simulink model "project4"  (R2023b)
settings: Solver=VariableStepAuto  StartTime=0.0  StopTime=10.0  RelTol=1e-3
undefined symbols (not defined in the file or in its folder): Kd, Ki, Kp
settings Model: Creator=mfb36  LastModifiedBy=mfb36

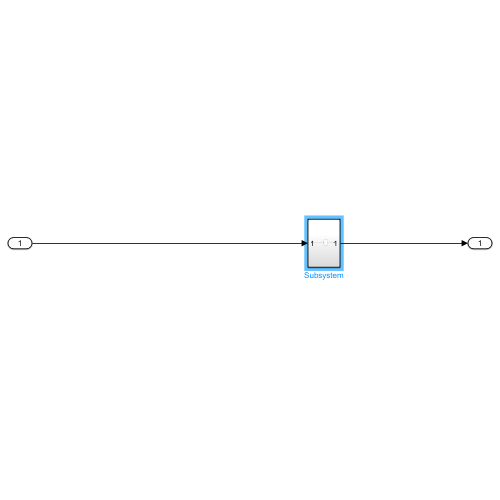
[thumbnail: Simulink's stored preview of the top-level diagram]
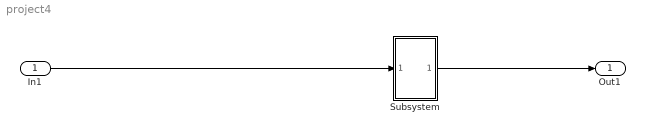
== system project4 ==
  In1 : Inport
  Subsystem : Subsystem
  Out1 : Outport
  wires:
  In1/1 -> Subsystem/1(In1)
  Subsystem/1(Out1) -> Out1/1

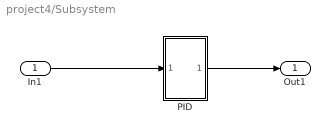
== system project4/Subsystem ==
  In1 : Inport
  PID : Subsystem
  Out1 : Outport
  wires:
  In1/1 -> PID/1(Error)
  PID/1(Control Action) -> Out1/1

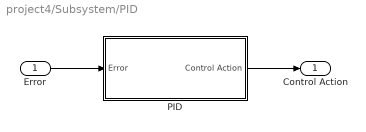
== system project4/Subsystem/PID ==
  Error : Inport
  PID : Subsystem
  Control Action : Outport
  wires:
  Error/1 -> PID/1(Error)
  PID/1(Control Action) -> Control Action/1

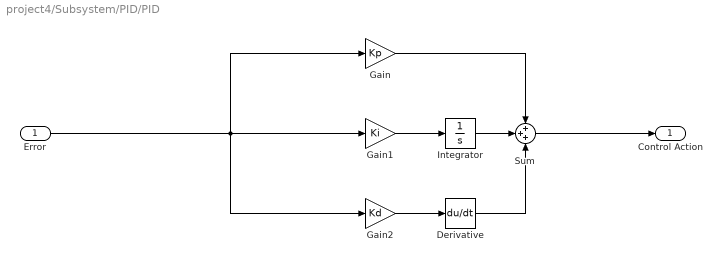
== system project4/Subsystem/PID/PID ==
  Error : Inport
  Derivative : Derivative
  Gain : Gain  Gain=Kp
  Gain1 : Gain  Gain=Ki
  Gain2 : Gain  Gain=Kd
  Integrator : Integrator
  Sum : Sum  Inputs=+++
  Control Action : Outport
  wires:
  Derivative/1 -> Sum/3
  Gain2/1 -> Derivative/1
  Error/1 -> Gain2/1, Gain/1, Gain1/1
  Gain1/1 -> Integrator/1
  Integrator/1 -> Sum/2
  Gain/1 -> Sum/1
  Sum/1 -> Control Action/1
